simulink model "MBLL"  (R2022a)
settings: Solver=VariableStepAuto  StartTime=0.0  StopTime=10.0  RelTol=1e-3
settings Model: Creator=mariodelossantos  LastModifiedBy=mariodelossantos

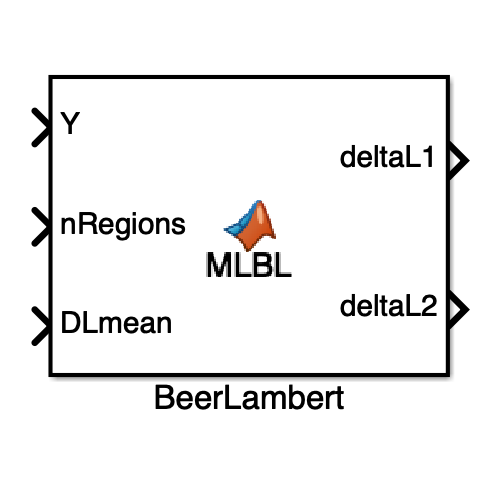
[thumbnail: Simulink's stored preview of the top-level diagram]
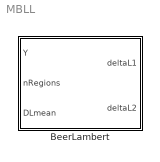
== system MBLL ==
  BeerLambert : MATLAB Function  TreatAsAtomicUnit=on

== matlab function MBLL/BeerLambert ==
  data: deltaL1 output; Y input; nRegions input; DLmean input; deltaL2 output
function [deltaL1,deltaL2]   = MLBL(Y, nRegions, DLmean)

%Molar extinction coefficients 
%Considering the wavelengths of the STak implentation, we need to use
% 780nm and 850nm

%780nm = [735.8251 1104.715];
%850nm = [1159.306 785.8993];
e_coefficients = [735.8251 1104.715;
                    1159.306 785.8993];

% https://mail.nmr.mgh.harvard.edu/pipermail//homer-users/2006-July/000124.html
%Differential Path Lenght
%NOTE: need to confirm this, I'm taking the values from an old
%implementation
DPF = [10.3; 8.4];

%Distance; this is an assumption of 3cm
Distance = 3;

%Using simulink is not possible to have a dynamic matrix that we can
%iterate based on the nRegions variable, but you could easly replace the
%number of regions in the variable "Regions" according your needs
DL1 = zeros(nRegions,1);
DL2 = zeros(nRegions,1);
%B = zeros(nRegions, nRegions);

%Divide the Lambdas (Not generalized yet)
DL1(1,1) = Y(1,1);
DL2(1,1) = Y(1,2);
DL1(2,1) = Y(2,1);
DL2(2,1) = Y(2,2);

A = [e_coefficients(1, 1)*Distance*DPF(1), e_coefficients(1, 2)*Distance*DPF(1);...
    e_coefficients(2, 1)*Distance*DPF(2), e_coefficients(2, 1)*Distance*DPF(2)];

deltaL1 = (-1)*log((DL1(:,1))/DLmean(1, 1));
deltaL2 = (-1)*log((DL2(:,1))/DLmean(1, 2));



Hemodynamics = linsolve(A, [deltaL1; deltaL2])' * (10^5);
